simulink model "pendulum_model_2015a"  (R2017b)
settings: Solver=ode45  StartTime=0.0  StopTime=20  RelTol=1e-3
values from neighbouring files (symbols this model uses):
  A_MAT = [0 0 1 0;0 0 0 1;A31 A32 A33 A34;A41 A42 A43 A44]    [Furuta233.m]    (also in Furuta_.m = [0 0 1 0;0 0 0 1;0 H1 H2 H3;0 H4 H5 H6]; Furuta_Template.m = [0 0 1 0;0 0 0 1;0 H1 H2 H3;0 H4 H5 H6]; Real_parameters.m = [0 0 1 0;0 0 0 1;0 24.4662 -0.0062 -0.0664;0 65.7367 -0.0051)
  b1 = 1*10^-4    (= 0.0001)    [Furuta233.m]    (also in Furuta_.m; Furuta_Template.m; Real_parameters.m)
  B_MAT = [0;0;B31;B41]    [Furuta233.m]    (also in Furuta_.m = [0;0;H7;H8]; Furuta_Template.m = [0;0;H7;H8]; Real_parameters.m = [0;0;3.2;3.1])
  C1 = -km/Lm    (= -18)    [Furuta233.m]    (also in Furuta_.m = -km/Lm; Furuta_Template.m = -km/Lm; Real_parameters.m)
  C2 = -Rm/Lm    (= -1560)    [Furuta233.m]    (also in Furuta_.m = -Rm/Lm; Furuta_Template.m = -Rm/Lm; Real_parameters.m)
  C3 = 1/Lm    (= 200)    [Furuta233.m]    (also in Furuta_.m = 1/Lm; Furuta_Template.m = 1/Lm; Real_parameters.m)
  C4 = km    (= 0.09)    [Furuta233.m]    (also in Furuta_.m = Km; Furuta_Template.m = Km; Real_parameters.m)
  C_MAT = [1 0 0 0;0 1 0 0]    [Furuta233.m]    (also in Furuta_.m = [1 1 0 0]; Furuta_Template.m = [1 1 0 0]; Real_parameters.m)
  E0 = 0.05    [Furuta233.m]    (also in Real_parameters.m = 0)
  F_MAT = -lqr(A_MAT,B_MAT,Q,R)    [Furuta233.m]    (also in Real_parameters.m = -[0.16 -320 1.3 -16])
  g = 9.81    [Furuta233.m]    (also in Furuta_.m; Furuta_Template.m; Real_parameters.m)
  J0 = J1 + (m1*((l1)^2)) + m2*((L1)^2)    (= 0.0373463)    [Furuta233.m]    (also in Furuta_.m; Furuta_Template.m; Real_parameters.m = 0.00503321266673)
  J2 = J2_1+(m2*((l2)^2))    (= 0.0055328)    [Furuta233.m]    (also in Furuta_.m; Furuta_Template.m; Real_parameters.m = 0.0020831968)
  K_swing = 0.1    [Furuta233.m]    (also in Real_parameters.m = -100)
  L1 = 0.278    [Furuta233.m]    (also in Furuta_.m; Furuta_Template.m; Real_parameters.m = sqrt(J1h/m1))
  l2 = 0.148    [Furuta233.m]    (also in Furuta_.m; Furuta_Template.m; Real_parameters.m = sqrt(J2/m2))
  L_MAT = -place(A_MAT',C_MAT',10*Closed_Loop_Poles)'    [Furuta233.m]    (also in Real_parameters.m = place(A_MAT',C_MAT',[12*Closed_Loop_Poles(1) 12*Closed_Loop_)
  m2 = 0.075    [Furuta233.m]    (also in Furuta_.m; Furuta_Template.m; Real_parameters.m = 0.049)
  xi = [0 0.1 0 0]    [Real_parameters.m]
libraries: simulink x1
settings Model: Creator=mectw  LastModifiedBy=lenovo
settings OptimizationCC: LifeSpan=inf
settings DebuggingCC: SFExecutionAtInitializationDiag=none
settings HardwareCC: ProdBitPerSizeT=32  ProdBitPerPtrDiffT=32  ProdWordSize=32  ProdHWDeviceType=Specified
settings CodeAppCC: StateflowObjectComments=on

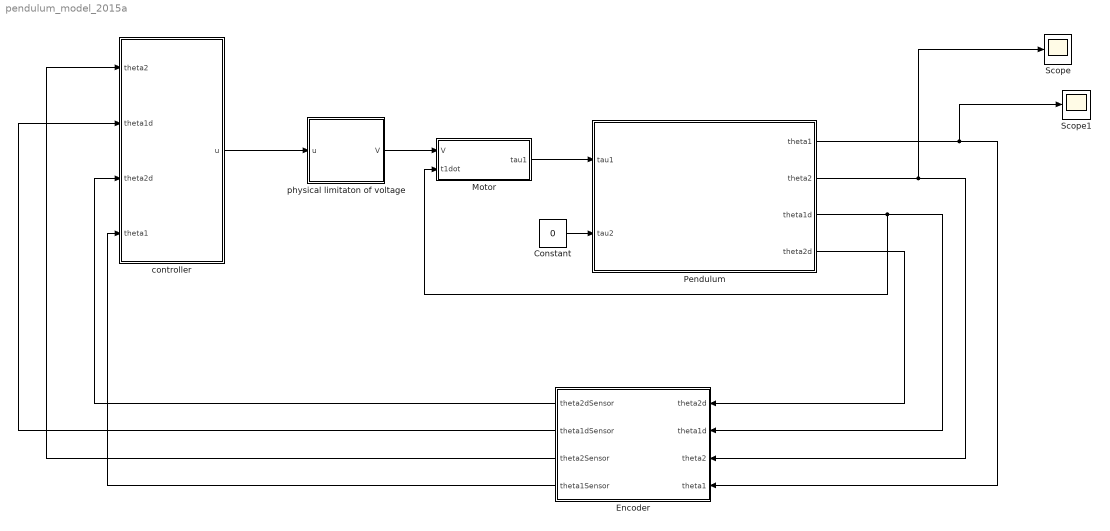
== system pendulum_model_2015a ==
  Constant : Constant  Value=0
  Encoder : Subsystem
  Motor : Subsystem
  Pendulum : Subsystem
  Scope : Scope
  Scope1 : Scope
  controller : Subsystem
  physical limitaton of voltage : Subsystem
  wires:
  Pendulum/1(theta1) -> Scope1/1, Encoder/4(theta1)
  Pendulum/2(theta2) -> Scope/1, Encoder/3(theta2)
  Pendulum/3(theta1d) -> Motor/2(t1dot), Encoder/2(theta1d)
  Pendulum/4(theta2d) -> Encoder/1(theta2d)
  controller/1(u) -> physical limitaton of voltage/1(u)
  physical limitaton of voltage/1(V) -> Motor/1(V)
  Motor/1(tau1) -> Pendulum/1(tau1)
  Constant/1 -> Pendulum/2(tau2)
  Encoder/4(theta1Sensor) -> controller/4(theta1)
  Encoder/3(theta2Sensor) -> controller/1(theta2)
  Encoder/2(theta1dSensor) -> controller/2(theta1d)
  Encoder/1(theta2dSensor) -> controller/3(theta2d)

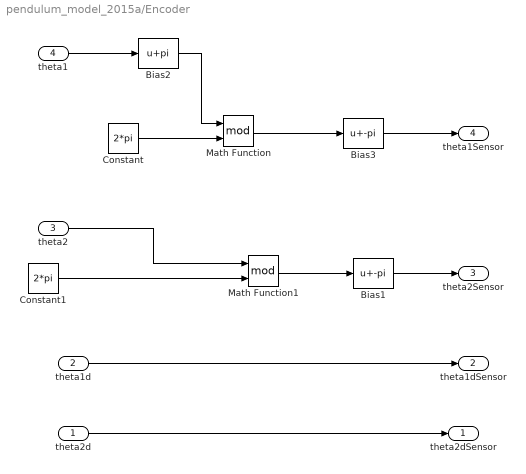
== system pendulum_model_2015a/Encoder ==
  theta2d : Inport
  theta1d : Inport  Port=2
  theta2 : Inport  Port=3
  theta1 : Inport  Port=4
  Bias1 : Bias  Bias=-pi
  Bias2 : Bias  Bias=pi
  Bias3 : Bias  Bias=-pi
  Constant : Constant  Value=2*pi
  Constant1 : Constant  Value=2*pi
  Math Function : Math  Operator=mod  SaturateOnIntegerOverflow=on
  Math Function1 : Math  Operator=mod  SaturateOnIntegerOverflow=on
  theta2dSensor : Outport
  theta1dSensor : Outport  Port=2
  theta2Sensor : Outport  Port=3
  theta1Sensor : Outport  Port=4
  wires:
  theta1d/1 -> theta1dSensor/1
  theta2d/1 -> theta2dSensor/1
  Constant/1 -> Math Function/2
  Constant1/1 -> Math Function1/2
  theta2/1 -> Math Function1/1
  Math Function1/1 -> Bias1/1
  Bias1/1 -> theta2Sensor/1
  theta1/1 -> Bias2/1
  Bias2/1 -> Math Function/1
  Math Function/1 -> Bias3/1
  Bias3/1 -> theta1Sensor/1

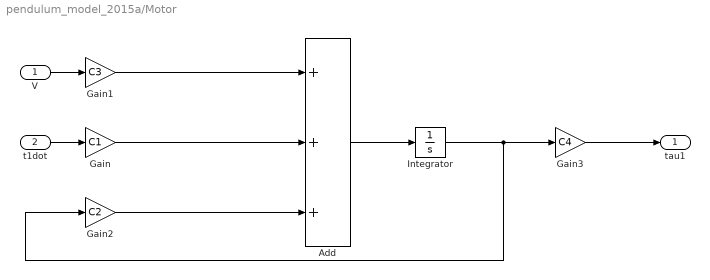
== system pendulum_model_2015a/Motor ==
  V : Inport
  t1dot : Inport  Port=2
  Add : Sum  Inputs=+++
  Gain : Gain  Gain=C1
  Gain1 : Gain  Gain=C3
  Gain2 : Gain  Gain=C2
  Gain3 : Gain  Gain=C4
  Integrator : Integrator
  tau1 : Outport
  wires:
  t1dot/1 -> Gain/1
  Gain1/1 -> Add/1
  Gain/1 -> Add/2
  Gain2/1 -> Add/3
  Add/1 -> Integrator/1
  Integrator/1 -> Gain3/1, Gain2/1
  Gain3/1 -> tau1/1
  V/1 -> Gain1/1

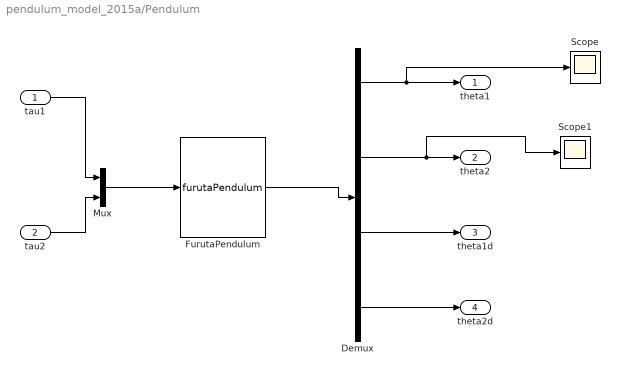
== system pendulum_model_2015a/Pendulum ==
  tau1 : Inport
  tau2 : Inport  Port=2
  Demux : Demux
  FurutaPendulum : S-Function  FunctionName=furutaPendulum  Parameters=J0, J2, m2, L1, l2, b1, b2, g, xi  SFunctionDeploymentMode=off  EnableBusSupport=off  mask{J0=J0, J2=J2, m2=m2, L1=L1, l2=l2, b1=b1, g=g, xi=[xi]}
      mask prompts: J0 "J0Hat"; J2 "J2Hat"
      mask Display: disp('FURUTA\nPENDULUM\n\nIn:[Tau1;Tau2]\nOut:x')
  Mux : Mux  Inputs=2
  Scope : Scope
  Scope1 : Scope
  theta1 : Outport
  theta2 : Outport  Port=2
  theta1d : Outport  Port=3
  theta2d : Outport  Port=4
  wires:
  tau1/1 -> Mux/1
  tau2/1 -> Mux/2
  FurutaPendulum/1 -> Demux/1
  Demux/1 -> Scope/1, theta1/1
  Demux/3 -> theta1d/1
  Demux/4 -> theta2d/1
  Mux/1 -> FurutaPendulum/1
  Demux/2 -> Scope1/1, theta2/1

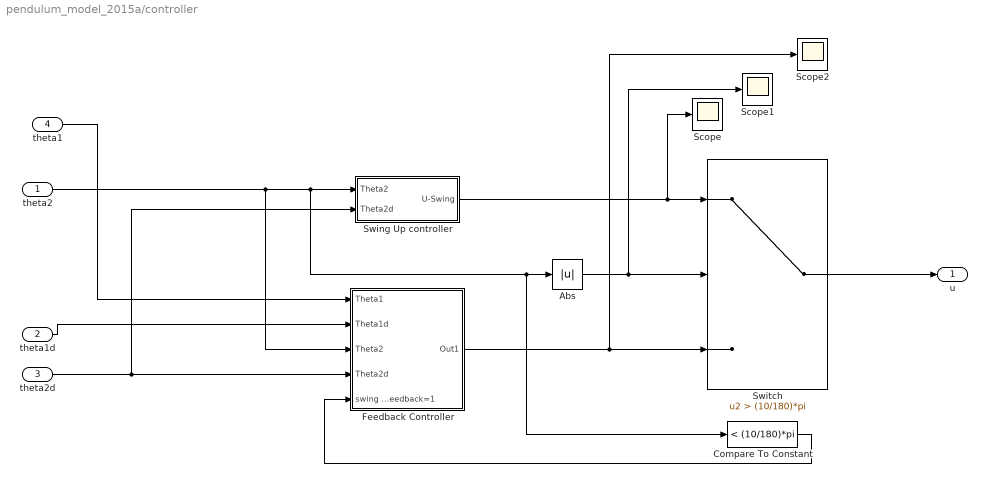
== system pendulum_model_2015a/controller ==
  theta2 : Inport
  theta1d : Inport  Port=2
  theta2d : Inport  Port=3
  theta1 : Inport  Port=4
  Abs : Abs
  Compare To Constant : simulink/Logic and Bit Operations/Compare To Constant  relop=<  const=(10/180)*pi  OutDataTypeStr=boolean
  Feedback Controller : Subsystem
  Scope : Scope
  Scope1 : Scope
  Scope2 : Scope
  Swing Up controller : Subsystem
  Switch : Switch  Criteria=u2 > Threshold  Threshold=(10/180)*pi
  u : Outport
  wires:
  theta2d/1 -> Feedback Controller/4("Theta2d "), Swing Up controller/2("Theta2d ")
  Feedback Controller/1(Out1) -> Scope2/1, Switch/3
  Abs/1 -> Scope1/1, Switch/2
  Switch/1 -> u/1
  Swing Up controller/1("U-Swing ") -> Scope/1, Switch/1
  theta1d/1 -> Feedback Controller/2("Theta1d ")
  theta2/1 -> Feedback Controller/3(Theta2), Compare To Constant/1, Abs/1, Swing Up controller/1("Theta2 ")
  theta1/1 -> Feedback Controller/1("Theta1 ")
  Compare To Constant/1 -> Feedback Controller/5("swing Up=0,feedback=1 ")

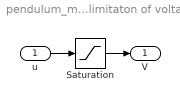
== system pendulum_model_2015a/physical limitaton of voltage ==
  u : Inport
  Saturation : Saturate  UpperLimit=10  LowerLimit=-10
  V : Outport
  wires:
  u/1 -> Saturation/1
  Saturation/1 -> V/1

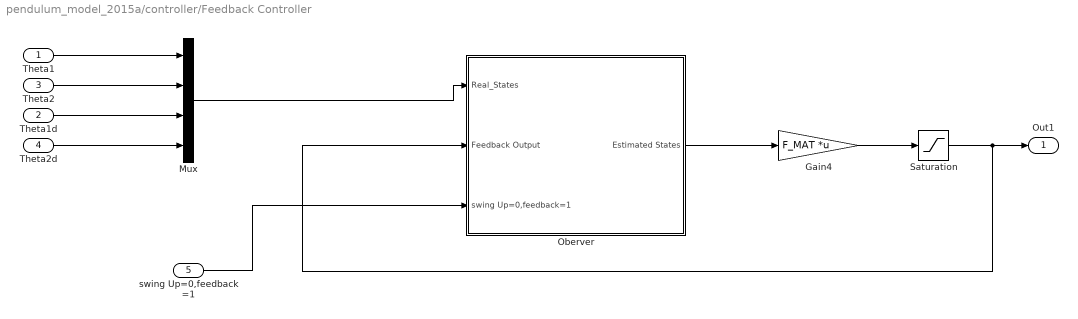
== system pendulum_model_2015a/controller/Feedback Controller ==
  "Theta1 " : Inport
  "Theta1d " : Inport  Port=2
  Theta2 : Inport  Port=3
  "Theta2d " : Inport  Port=4
  "swing Up=0,feedback=1 " : Inport  Port=5
  Gain4 : Gain  Gain=F_MAT  Multiplication=Matrix(K*u)
  Mux : Mux
  "Oberver " : Subsystem
  Saturation : Saturate
  Out1 : Outport
  wires:
  "Theta1d "/1 -> Mux/3
  Mux/1 -> "Oberver "/1(Real_States)
  "Theta2d "/1 -> Mux/4
  "Theta1 "/1 -> Mux/1
  Theta2/1 -> Mux/2
  Gain4/1 -> Saturation/1
  Saturation/1 -> "Oberver "/2(Feedback Output), Out1/1
  "swing Up=0,feedback=1 "/1 -> "Oberver "/3("swing Up=0,feedback=1 ")
  "Oberver "/1(Estimated States) -> Gain4/1

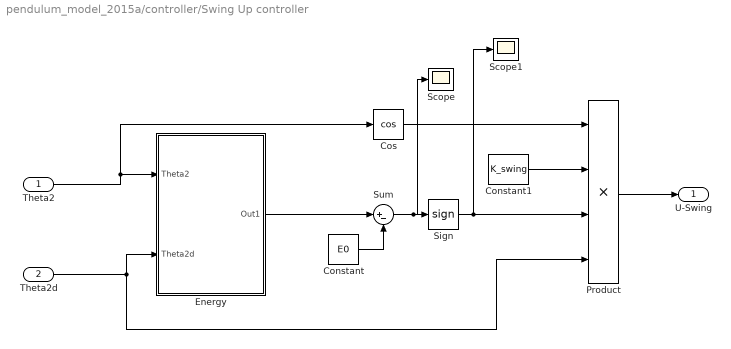
== system pendulum_model_2015a/controller/Swing Up controller ==
  "Theta2 " : Inport
  "Theta2d " : Inport  Port=2
  Constant : Constant  Value=E0
  Constant1 : Constant  Value=K_swing
  Cos : Trigonometry  Operator=cos
  Energy : Subsystem
  Product : Product  Inputs=4
  Scope : Scope
  Scope1 : Scope
  Sign : Signum
  Sum : Sum  Inputs=|+-
  "U-Swing " : Outport
  wires:
  "Theta2 "/1 -> Cos/1, Energy/1("Theta2 ")
  "Theta2d "/1 -> Energy/2("Theta2d "), Product/4
  Energy/1(Out1) -> Sum/1
  Cos/1 -> Product/1
  Constant/1 -> Sum/2
  Sum/1 -> Scope/1, Sign/1
  Sign/1 -> Scope1/1, Product/3
  Constant1/1 -> Product/2
  Product/1 -> "U-Swing "/1

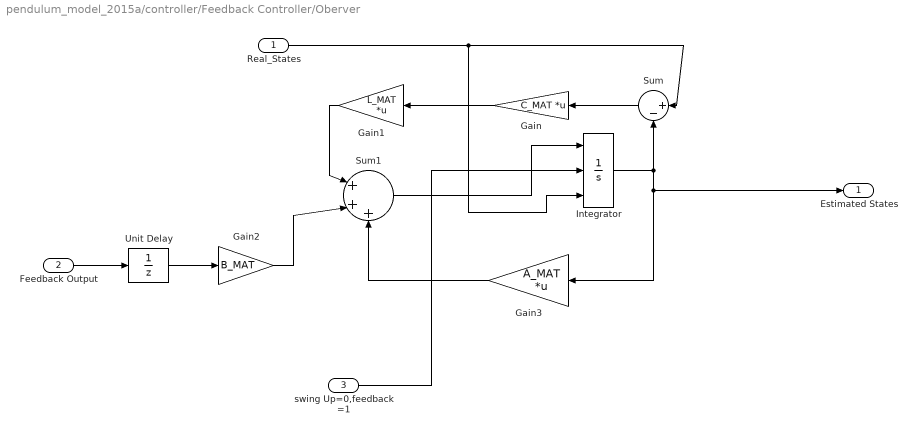
== system pendulum_model_2015a/controller/Feedback Controller/Oberver  ==
  Real_States : Inport
  Feedback Output : Inport  Port=2
  "swing Up=0,feedback=1 " : Inport  Port=3  OutDataTypeStr=boolean
  Gain : Gain  Gain=C_MAT  Multiplication=Matrix(K*u)
  Gain1 : Gain  Gain=L_MAT  Multiplication=Matrix(K*u)
  Gain2 : Gain  Gain=B_MAT
  Gain3 : Gain  Gain=A_MAT  Multiplication=Matrix(K*u)
  Integrator : Integrator  ExternalReset=either  InitialConditionSource=external
  Sum : Sum  Inputs=|+-
  Sum1 : Sum  Inputs=|+++
  Unit Delay : UnitDelay  SampleTime=-1
  Estimated States : Outport
  wires:
  Real_States/1 -> Integrator/3, Sum/1
  Sum/1 -> Gain/1
  Gain/1 -> Gain1/1
  Gain1/1 -> Sum1/1
  Sum1/1 -> Integrator/1
  Integrator/1 -> Gain3/1, Estimated States/1, Sum/2
  Gain3/1 -> Sum1/3
  Gain2/1 -> Sum1/2
  Unit Delay/1 -> Gain2/1
  Feedback Output/1 -> Unit Delay/1
  "swing Up=0,feedback=1 "/1 -> Integrator/2

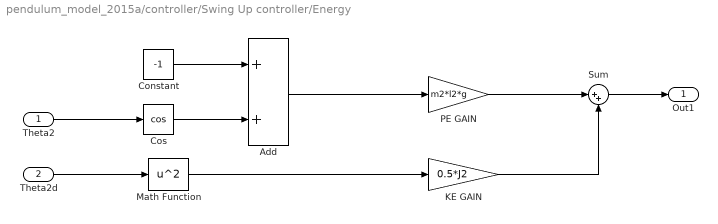
== system pendulum_model_2015a/controller/Swing Up controller/Energy ==
  "Theta2 " : Inport
  "Theta2d " : Inport  Port=2
  Add : Sum
  Constant : Constant  Value=-1
  Cos : Trigonometry  Operator=cos
  KE GAIN : Gain  Gain=0.5*J2
  Math Function : Math  Operator=square  SaturateOnIntegerOverflow=on
  PE GAIN : Gain  Gain=m2*l2*g
  Sum : Sum  Inputs=|++
  Out1 : Outport
  wires:
  "Theta2 "/1 -> Cos/1
  Constant/1 -> Add/1
  Cos/1 -> Add/2
  Add/1 -> PE GAIN/1
  "Theta2d "/1 -> Math Function/1
  PE GAIN/1 -> Sum/1
  Math Function/1 -> KE GAIN/1
  KE GAIN/1 -> Sum/2
  Sum/1 -> Out1/1
